simulink model "sl_subsys_fcncallerr14"  (Simulink 7.6)
settings: Solver=FixedStepDiscrete  StartTime=0.0  StopTime=10.0  RelTol=1e-3
settings Model: Creator=The MathWorks Inc.
settings DataIOCC: SaveState=on
settings DebuggingCC: UnderspecifiedInitializationDetection=Simplified  StrictBusMsg=ErrorOnBusTreatedAsVector
settings SFSimCC: SimParseCustomCode=off

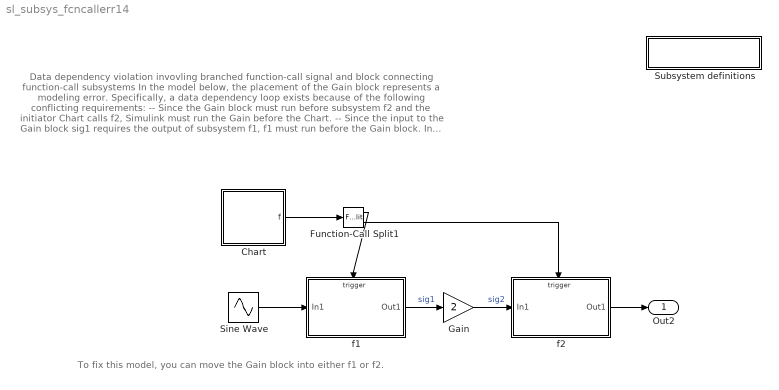
== system sl_subsys_fcncallerr14 ==
  note: To fix this model, you can move the Gain block into either f1 or f2.
  note: Data dependency violation invovling branched function-call signal and block
      | connecting function-call subsystems
      |
      | In the model below, the placement of the Gain block represents a modeling error.
      | Specifically, a data dependency loop exists because of the following conflicting
      | requirements:
      | -- Since the Gain block must run before subsystem f2 and the initiator Chart
      | calls f2, Simulink must run the Gain before the Chart.
      | -- Since the input to the Gain block sig1 requires the output of subsystem f1,
      | f1 must run before the Gain block. In turn, the initiator Chart must call f1 before
      | the Gain block runs.
  " Subsystem definitions" : Subsystem
      settings: OpenFcn=helpview([matlabroot,'/toolbox/simulink/simdemos/simfeatures/html/sl_subsys_definitions.html']);
      mask Display: disp('Subsystem\ndefinitions')
  Chart : Stateflow chart  TreatAsAtomicUnit=on
  Function-Call Split1 : FunctionCallSplit
  Gain : Gain  Gain=2
  Sine Wave : Sin  SampleTime=1
  f1 : Subsystem  TreatAsAtomicUnit=on
  f2 : Subsystem  TreatAsAtomicUnit=on
  Out2 : Outport
  wires:
  Chart/1(f) -> Function-Call Split1/1
  f2/1(Out1) -> Out2/1
  Function-Call Split1/1 -> f1/Trigger
  Function-Call Split1/2 -> f2/Trigger
  f1/1(Out1) -> Gain/1  "sig1"
  Sine Wave/1 -> f1/1(In1)
  Gain/1 -> f2/1(In1)  "sig2"

== system sl_subsys_fcncallerr14/ Subsystem definitions ==

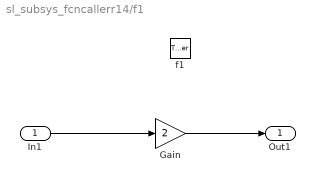
== system sl_subsys_fcncallerr14/f1 ==
  In1 : Inport
  f1 : TriggerPort  TriggerType=function-call  SampleTimeType=periodic
  Gain : Gain  Gain=2
  Out1 : Outport  InitialOutput=1/1000
      settings: AttributesFormatString=%<OutputWhenDisabled>: %<InitialOutput>
  wires:
  Gain/1 -> Out1/1
  In1/1 -> Gain/1

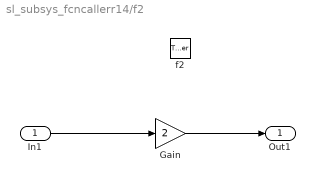
== system sl_subsys_fcncallerr14/f2 ==
  In1 : Inport
  f2 : TriggerPort  TriggerType=function-call  SampleTimeType=periodic
  Gain : Gain  Gain=2
  Out1 : Outport  InitialOutput=1/1000
      settings: AttributesFormatString=%<OutputWhenDisabled>: %<InitialOutput>
  wires:
  In1/1 -> Gain/1
  Gain/1 -> Out1/1

== stateflow chart Chart ==
  state one/
    entry: f;
  state two/
    entry: f;
  one -> two
  two -> one
  (default) -> one
  events: f output FUNCTION_CALL_EVENT
